simulink library "INP_SPDWHL_ManOver"  (R2024b)
settings: Solver=VariableStepAuto  StartTime=0.0  StopTime=10.0  RelTol=1e-3
undefined symbols (not defined in the file): INP_SPDWHL_p_SwtSpdWhlFrLeMan_na, INP_SPDWHL_p_SwtSpdWhlFrRiMan_na, INP_SPDWHL_p_SwtSpdWhlReLeMan_na, INP_SPDWHL_p_SwtSpdWhlReRiMan_na, INP_SPDWHL_s_SpdWhlFrLeMan_radps, INP_SPDWHL_s_SpdWhlFrRiMan_radps, INP_SPDWHL_s_SpdWhlLoLimFrLe_radps, INP_SPDWHL_s_SpdWhlLoLimFrRi_radps, INP_SPDWHL_s_SpdWhlLoLimReLe_radps, INP_SPDWHL_s_SpdWhlLoLimReRi_radps, INP_SPDWHL_s_SpdWhlReLeMan_radps, INP_SPDWHL_s_SpdWhlReRiMan_radps, INP_SPDWHL_s_SpdWhlUpLimFrLe_radps, INP_SPDWHL_s_SpdWhlUpLimFrRi_radps, INP_SPDWHL_s_SpdWhlUpLimReLe_radps, INP_SPDWHL_s_SpdWhlUpLimReRi_radps
libraries: simulink x4
settings Model: Creator=blatak  LastModifiedBy=jmbsp

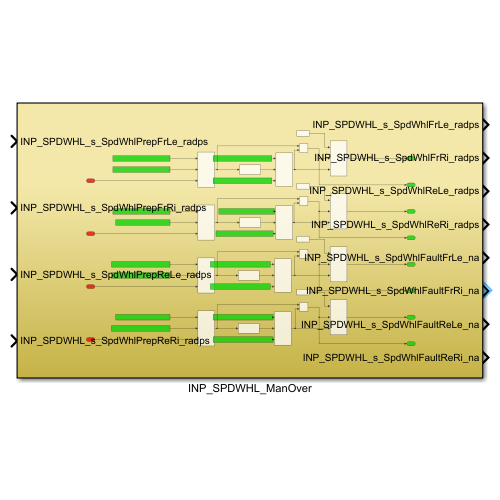
[thumbnail: Simulink's stored preview of the top-level diagram]
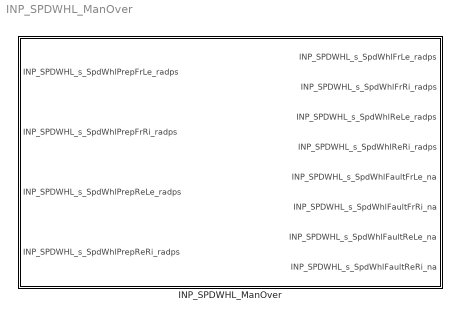
== system INP_SPDWHL_ManOver ==
  INP_SPDWHL_ManOver : Subsystem

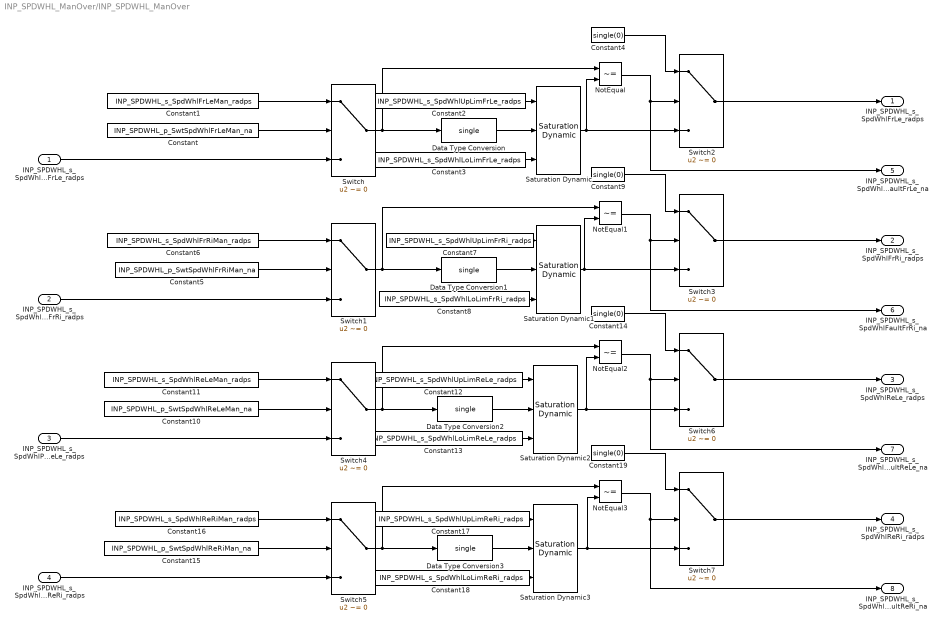
== system INP_SPDWHL_ManOver/INP_SPDWHL_ManOver ==
  INP_SPDWHL_s_SpdWhlPrepFrLe_radps : Inport
  INP_SPDWHL_s_SpdWhlPrepFrRi_radps : Inport  Port=2
  INP_SPDWHL_s_SpdWhlPrepReLe_radps : Inport  Port=3
  INP_SPDWHL_s_SpdWhlPrepReRi_radps : Inport  Port=4
  Constant : Constant  Description=|  Value=INP_SPDWHL_p_SwtSpdWhlFrLeMan_na
      | Switch for manual override of the longitudinal acceleration value, if 1 instead the measured 
      | value the INP_IMU_p_ALgtVehMan_mps2 is used
  Constant1 : Constant  Description=|  Value=INP_SPDWHL_s_SpdWhlFrLeMan_radps
      | Value for longitudinal acceleration, which is used if the INP_IMU_p_SwtAXxxVehMan_na
      | is set to 1 instead of the measured value
  Constant10 : Constant  Description=|  Value=INP_SPDWHL_p_SwtSpdWhlReLeMan_na
      | Switch for manual override of the longitudinal acceleration value, if 1 instead the measured 
      | value the INP_IMU_p_ALgtVehMan_mps2 is used
  Constant11 : Constant  Description=|  Value=INP_SPDWHL_s_SpdWhlReLeMan_radps
      | Value for longitudinal acceleration, which is used if the INP_IMU_p_SwtAXxxVehMan_na
      | is set to 1 instead of the measured value
  Constant12 : Constant  Description=Upper saturation limit for longitudinal acceleration  Value=INP_SPDWHL_s_SpdWhlUpLimReLe_radps
  Constant13 : Constant  Description=Lower saturation limit for longitudinal acceleration  Value=INP_SPDWHL_s_SpdWhlLoLimReLe_radps
  Constant{4,9,14,19} (4 alike) : Constant  Value=single(0)
  Constant15 : Constant  Description=|  Value=INP_SPDWHL_p_SwtSpdWhlReRiMan_na
      | Switch for manual override of the longitudinal acceleration value, if 1 instead the measured 
      | value the INP_IMU_p_ALgtVehMan_mps2 is used
  Constant16 : Constant  Description=|  Value=INP_SPDWHL_s_SpdWhlReRiMan_radps
      | Value for longitudinal acceleration, which is used if the INP_IMU_p_SwtAXxxVehMan_na
      | is set to 1 instead of the measured value
  Constant17 : Constant  Description=Upper saturation limit for longitudinal acceleration  Value=INP_SPDWHL_s_SpdWhlUpLimReRi_radps
  Constant18 : Constant  Description=Lower saturation limit for longitudinal acceleration  Value=INP_SPDWHL_s_SpdWhlLoLimReRi_radps
  Constant2 : Constant  Description=Upper saturation limit for longitudinal acceleration  Value=INP_SPDWHL_s_SpdWhlUpLimFrLe_radps
  Constant3 : Constant  Description=Lower saturation limit for longitudinal acceleration  Value=INP_SPDWHL_s_SpdWhlLoLimFrLe_radps
  Constant5 : Constant  Description=|  Value=INP_SPDWHL_p_SwtSpdWhlFrRiMan_na
      | Switch for manual override of the longitudinal acceleration value, if 1 instead the measured 
      | value the INP_IMU_p_ALgtVehMan_mps2 is used
  Constant6 : Constant  Description=|  Value=INP_SPDWHL_s_SpdWhlFrRiMan_radps
      | Value for longitudinal acceleration, which is used if the INP_IMU_p_SwtAXxxVehMan_na
      | is set to 1 instead of the measured value
  Constant7 : Constant  Description=Upper saturation limit for longitudinal acceleration  Value=INP_SPDWHL_s_SpdWhlUpLimFrRi_radps
  Constant8 : Constant  Description=Lower saturation limit for longitudinal acceleration  Value=INP_SPDWHL_s_SpdWhlLoLimFrRi_radps
  Data Type Conversion{,1..3} (4 alike) : DataTypeConversion  OutDataTypeStr=single  SaturateOnIntegerOverflow=off  RndMeth=Floor
  NotEqual{,1..3} (4 alike) : RelationalOperator  Operator=~=  OutDataTypeStr=boolean  RndMeth=Simplest  InputSameDT=off
  Saturation Dynamic{,1..3} (4 alike) : simulink/Discontinuities/Saturation Dynamic  OutMin=[]  OutMax=[]  OutDataTypeStr=Inherit: Same as second input  OutDataType=fixdt(1, 16)  OutScaling=2^-10  DoSatur=off
  Switch{,1..7} (8 alike) : Switch  Criteria=u2 ~= 0  SaturateOnIntegerOverflow=off  InputSameDT=off
  INP_SPDWHL_s_SpdWhlFrLe_radps : Outport
  INP_SPDWHL_s_SpdWhlFrRi_radps : Outport  Port=2
  INP_SPDWHL_s_SpdWhlReLe_radps : Outport  Port=3
  INP_SPDWHL_s_SpdWhlReRi_radps : Outport  Port=4
  INP_SPDWHL_s_SpdWhlFaultFrLe_na : Outport  Port=5
  INP_SPDWHL_s_SpdWhlFaultFrRi_na : Outport  Port=6
  INP_SPDWHL_s_SpdWhlFaultReLe_na : Outport  Port=7
  INP_SPDWHL_s_SpdWhlFaultReRi_na : Outport  Port=8
  wires:
  Switch4/1 -> NotEqual2/1, Data Type Conversion2/1
  Constant/1 -> Switch/2
  INP_SPDWHL_s_SpdWhlPrepReLe_radps/1 -> Switch4/3
  Constant19/1 -> Switch7/1
  Saturation Dynamic2/1 -> Switch6/3, NotEqual2/2
  Constant8/1 -> Saturation Dynamic1/3
  Constant16/1 -> Switch5/1
  Data Type Conversion3/1 -> Saturation Dynamic3/2
  Saturation Dynamic3/1 -> Switch7/3, NotEqual3/2
  Constant1/1 -> Switch/1
  Constant4/1 -> Switch2/1
  NotEqual1/1 -> INP_SPDWHL_s_SpdWhlFaultFrRi_na/1, Switch3/2
  NotEqual3/1 -> INP_SPDWHL_s_SpdWhlFaultReRi_na/1, Switch7/2
  Saturation Dynamic1/1 -> Switch3/3, NotEqual1/2
  Constant14/1 -> Switch6/1
  Switch/1 -> NotEqual/1, Data Type Conversion/1
  Constant2/1 -> Saturation Dynamic/1
  Constant5/1 -> Switch1/2
  Switch7/1 -> INP_SPDWHL_s_SpdWhlReRi_radps/1
  Constant15/1 -> Switch5/2
  Constant6/1 -> Switch1/1
  NotEqual/1 -> INP_SPDWHL_s_SpdWhlFaultFrLe_na/1, Switch2/2
  Saturation Dynamic/1 -> Switch2/3, NotEqual/2
  INP_SPDWHL_s_SpdWhlPrepFrLe_radps/1 -> Switch/3
  Switch2/1 -> INP_SPDWHL_s_SpdWhlFrLe_radps/1
  Constant10/1 -> Switch4/2
  Constant3/1 -> Saturation Dynamic/3
  Switch6/1 -> INP_SPDWHL_s_SpdWhlReLe_radps/1
  Constant12/1 -> Saturation Dynamic2/1
  Constant9/1 -> Switch3/1
  Constant13/1 -> Saturation Dynamic2/3
  Constant7/1 -> Saturation Dynamic1/1
  NotEqual2/1 -> INP_SPDWHL_s_SpdWhlFaultReLe_na/1, Switch6/2
  INP_SPDWHL_s_SpdWhlPrepFrRi_radps/1 -> Switch1/3
  Switch3/1 -> INP_SPDWHL_s_SpdWhlFrRi_radps/1
  Data Type Conversion2/1 -> Saturation Dynamic2/2
  Constant17/1 -> Saturation Dynamic3/1
  Switch1/1 -> NotEqual1/1, Data Type Conversion1/1
  INP_SPDWHL_s_SpdWhlPrepReRi_radps/1 -> Switch5/3
  Data Type Conversion/1 -> Saturation Dynamic/2
  Constant11/1 -> Switch4/1
  Data Type Conversion1/1 -> Saturation Dynamic1/2
  Switch5/1 -> NotEqual3/1, Data Type Conversion3/1
  Constant18/1 -> Saturation Dynamic3/3
